simulink model "assignment_R2018A"  (R2018a)
settings: Solver=VariableStepAuto  StartTime=0.0  StopTime=simulation_time
undefined symbols (not defined in the file or in its folder): a, A_BN_0, A_epsilon, A_i, a_m, C_d, dim, DiscIntNeverNeededParam, gm, gn, gsvi, gvali, hm, hn, hsvi, hvali, I, i, I_inv, k_bdot, k_d, k_p, m_max, max_momentum, max_torque, mu, nadir_vector, OMG, omg, phi_0, psi_0, q_0, q_c, R_e, rho_d, rho_s, sigma_e, theta, theta_0, w_0, w_e
libraries: sharedutil x4, simulink_extras x3, aerolibconvert2 x2, simulink x2, vrlib x1
(part 1 of 2)
settings Model: Creator=fcuzzocrea  LastModifiedBy=fcuzzocrea
settings SolverCC: ShapePreserveControl=EnableAll
settings OptimizationCC: DefaultParameterBehavior=Inlined  UseDivisionForNetSlopeComputation=on  UseFloatMulNetSlope=on  InlineInvariantSignals=on  PassReuseOutputArgsAs=Individual arguments  ZeroExternalMemoryAtStartup=off  ZeroInternalMemoryAtStartup=off  NoFixptDivByZeroProtection=on  EfficientFloat2IntCast=on  LifeSpan=1  OptimizeBlockOrder=speed  DifferentSizesBufferReuse=on
settings DebuggingCC: ParameterTunabilityLossMsg=error
settings HardwareCC: ProdBitPerInt=16  ProdBitPerPointer=16  ProdBitPerSizeT=16  ProdBitPerPtrDiffT=16  ProdLargestAtomicFloat=None  ProdWordSize=16  ProdLongLongMode=on  ProdHWDeviceType=STMicroelectronics->ST10/Super10  TargetBitPerLong=64  TargetBitPerPointer=64  TargetBitPerSizeT=64  TargetBitPerPtrDiffT=64  TargetLongLongMode=on  TargetIntDivRoundTo=Zero  TargetEndianess=LittleEndian  TargetWordSize=64  TargetHWDeviceType=MATLAB Host  ProdEqTarget=off
settings SFSimCC: MATLABDynamicMemAlloc=off
settings RTWCC: SystemTargetFile=ert.tlc  TemplateMakefile=ert_default_tmf  GenerateReport=on  RTWUseLocalCustomCode=on  IncludeHyperlinkInReport=on  LaunchReport=on  GenerateTraceInfo=on  GenerateTraceReport=on  GenerateTraceReportSl=on  GenerateTraceReportSf=on  GenerateTraceReportEml=on  GenerateCodeMetricsReport=on
settings CodeAppCC: ForceParamTrailComments=on  IgnoreCustomStorageClasses=off  MaxIdLength=128  OperatorAnnotations=on  SimulinkDataObjDesc=on  SFDataObjDesc=on  CustomSymbolStrGlobalVar=rt$N$M  CustomSymbolStrType=$N$M  CustomSymbolStrFcn=$N$M$F  CustomSymbolStrMacro=$N$M  InsertBlockDesc=on
settings ERTTargetCC: GenerateSampleERTMain=on  IncludeMdlTerminateFcn=off  CombineSignalStateStructs=on  SupportComplex=off  SupportContinuousTime=on  SupportNonInlinedSFcns=on  InlinedParameterPlacement=NonHierarchical  ERTCustomFileTemplate=example_file_process.tlc  ERTFilePackagingFormat=CompactWithDataFile

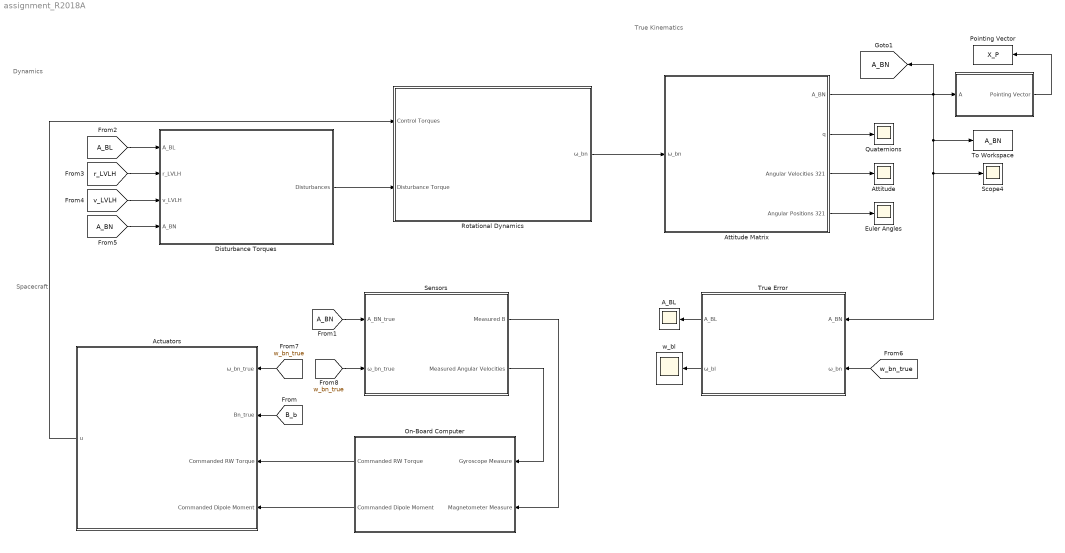
== system assignment_R2018A ==
  note: True Kinematics
  note: Dynamics
  note: Spacecraft
  " " : Subsystem
  " Sensors" : Subsystem
  A_BL : Scope
  Actuators : Subsystem
  Attitude : Scope
  Attitude Matrix : Subsystem
  Disturbance Torques : Subsystem
  Euler Angles : Scope
  On-Board Computer : Subsystem
  Pointing Vector : ToWorkspace  VariableName=X_P  SampleTime=-1
  Quaternions : Scope
  "Rotational Dynamics " : Subsystem
  Scope4 : Scope
  To Workspace : ToWorkspace  VariableName=A_BN  SampleTime=-1
  True Error : Subsystem
  w_bl : Scope
  tag scope: A_BN=global
  wires:
  [r_LVLH] -> Disturbance Torques/2(r_LVLH)
  " "/1("Pointing Vector ") -> Pointing Vector/1
  Attitude Matrix/4(Angular Positions 321) -> Euler Angles/1
  Attitude Matrix/2(q) -> Quaternions/1
  Attitude Matrix/1(A_BN) -> " "/1(A), To Workspace/1, Scope4/1, True Error/1(A_BN), [A_BN]
  [A_BL] -> Disturbance Torques/1(A_BL)
  Attitude Matrix/3(Angular Velocities 321) -> Attitude/1
  [A_BN] -> Disturbance Torques/4(A_BN)
  Disturbance Torques/1(Disturbances) -> "Rotational Dynamics "/2("Disturbance Torque ")
  [v_LVLH] -> Disturbance Torques/3(v_LVLH)
  " Sensors"/2(Measured Angular Velocities) -> On-Board Computer/1(Gyroscope Measure)
  " Sensors"/1(Measured B) -> On-Board Computer/2(Magnetometer Measure)
  True Error/1(A_BL) -> A_BL/1
  On-Board Computer/1(Commanded RW Torque) -> Actuators/3(Commanded RW Torque)
  On-Board Computer/2(Commanded Dipole Moment) -> Actuators/4(Commanded Dipole Moment)
  [B_b] -> Actuators/2(Bn_true)
  "Rotational Dynamics "/1(ω_bn) -> Attitude Matrix/1(ω_bn)
  [A_BN] -> " Sensors"/1(A_BN_true)
  [w_bn_true] -> True Error/2(ω_bn)
  [w_bn_true] -> Actuators/1(ω_bn_true)
  [w_bn_true] -> " Sensors"/2(ω_bn_true)
  Actuators/1(u) -> "Rotational Dynamics "/1(Control Torques)
  True Error/2(ω_bl) -> w_bl/1

== system assignment_R2018A/  ==
  A : Inport
  Constant3 : Constant  Value=[1; 0; 0]  VectorParams1D=off
  Math Function : Math  Operator=transpose  SaturateOnIntegerOverflow=on
  Product1 : Product  Multiplication=Matrix(*)
  "Pointing Vector " : Outport
  wires:
  Constant3/1 -> Product1/2
  Math Function/1 -> Product1/1
  A/1 -> Math Function/1
  Product1/1 -> "Pointing Vector "/1

== system assignment_R2018A/ Sensors ==
  A_BN_true : Inport
  ω_bn_true : Inport  Port=2
  Gyroscope : Subsystem
  Magnetometer : Subsystem
  Zero-Order Hold : ZeroOrderHold  SampleTime=-1
  Zero-Order Hold1 : ZeroOrderHold  SampleTime=-1
  Measured B : Outport
  Measured Angular Velocities : Outport  Port=2
  wires:
  A_BN_true/1 -> Magnetometer/1(A_BN)
  ω_bn_true/1 -> Gyroscope/1(ω_bn)
  Gyroscope/1(Angular Velocities) -> Zero-Order Hold/1
  Magnetometer/1(Magnetic Field) -> Zero-Order Hold1/1
  Zero-Order Hold/1 -> Measured Angular Velocities/1
  Zero-Order Hold1/1 -> Measured B/1

== system assignment_R2018A/Actuators ==
  ω_bn_true : Inport
  Bn_true : Inport  Port=2
  Commanded RW Torque : Inport  Port=3
  Commanded Dipole Moment : Inport  Port=4
  Magnetic Torquers : Subsystem
  Reaction Wheels : Subsystem
  Sum : Sum  Inputs=|++
  To Workspace1 : ToWorkspace  VariableName=control_torque  SampleTime=-1
  u : Outport
  wires:
  Reaction Wheels/1(Control Torque) -> Sum/1
  ω_bn_true/1 -> Reaction Wheels/1(w_bn)
  Commanded RW Torque/1 -> Reaction Wheels/2(Commanded Torque)
  Magnetic Torquers/1(Control Torque) -> Sum/2
  Commanded Dipole Moment/1 -> Magnetic Torquers/2(Commanded Dipole Moment)
  Bn_true/1 -> Magnetic Torquers/1(B)
  Sum/1 -> To Workspace1/1, u/1

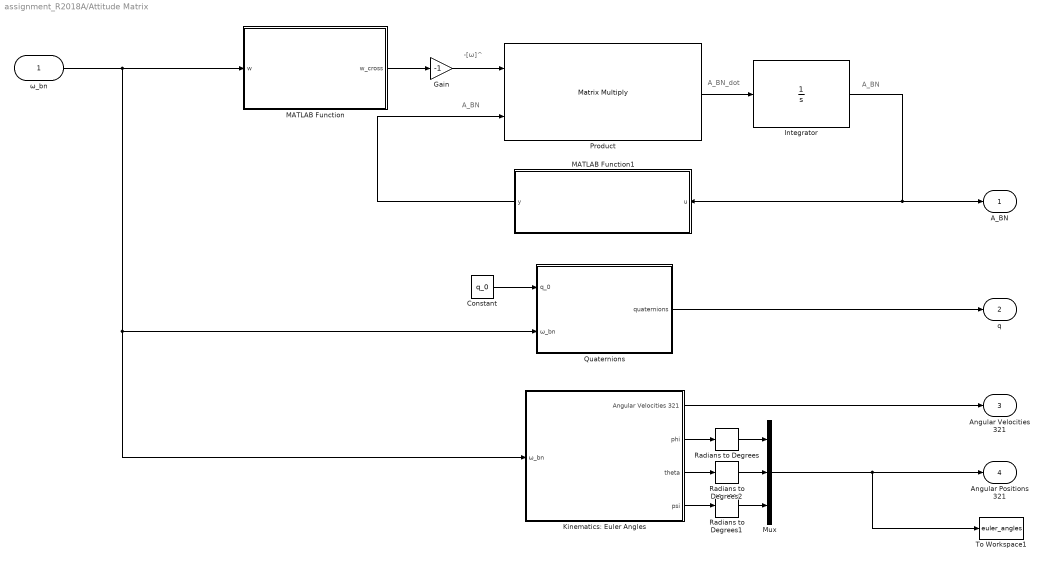
== system assignment_R2018A/Attitude Matrix ==
  note: -[ω]^
  note: A_BN_dot
  note: A_BN
  note: A_BN
  ω_bn : Inport  Unit=rad/s  PortDimensions=3
  Constant : Constant  Value=q_0
  Gain : Gain  Gain=-1
  Integrator : Integrator  InitialCondition=A_BN_0
  Kinematics: Euler Angles : Subsystem
  MATLAB Function : MATLAB Function  TreatAsAtomicUnit=on
  MATLAB Function1 : MATLAB Function  TreatAsAtomicUnit=on
  Mux : Mux  Inputs=3
  Product : Product  Multiplication=Matrix(*)
  Quaternions : Subsystem
  Radians to Degrees : simulink_extras/Transformations/Radians to Degrees
  Radians to Degrees1 : simulink_extras/Transformations/Radians to Degrees
  Radians to Degrees2 : simulink_extras/Transformations/Radians to Degrees
  To Workspace1 : ToWorkspace  VariableName=euler_angles  SampleTime=-1
  A_BN : Outport
  q : Outport  Port=2
  Angular Velocities 321 : Outport  Port=3
  Angular Positions 321 : Outport  Port=4
  wires:
  Product/1 -> Integrator/1
  MATLAB Function/1(w_cross) -> Gain/1
  Integrator/1 -> MATLAB Function1/1(u), A_BN/1
  ω_bn/1 -> MATLAB Function/1(w), Quaternions/2(ω_bn), Kinematics: Euler Angles/1(ω_bn)
  Kinematics: Euler Angles/1(Angular Velocities 321) -> Angular Velocities 321/1
  Kinematics: Euler Angles/3(theta) -> Radians to Degrees2/1
  Kinematics: Euler Angles/4(psi) -> Radians to Degrees1/1
  Kinematics: Euler Angles/2(phi) -> Radians to Degrees/1
  Gain/1 -> Product/1
  Quaternions/1(quaternions) -> q/1
  MATLAB Function1/1(y) -> Product/2
  Constant/1 -> Quaternions/1("q_0 ")
  Radians to Degrees/1 -> Mux/1
  Radians to Degrees2/1 -> Mux/2
  Radians to Degrees1/1 -> Mux/3
  Mux/1 -> To Workspace1/1, Angular Positions 321/1

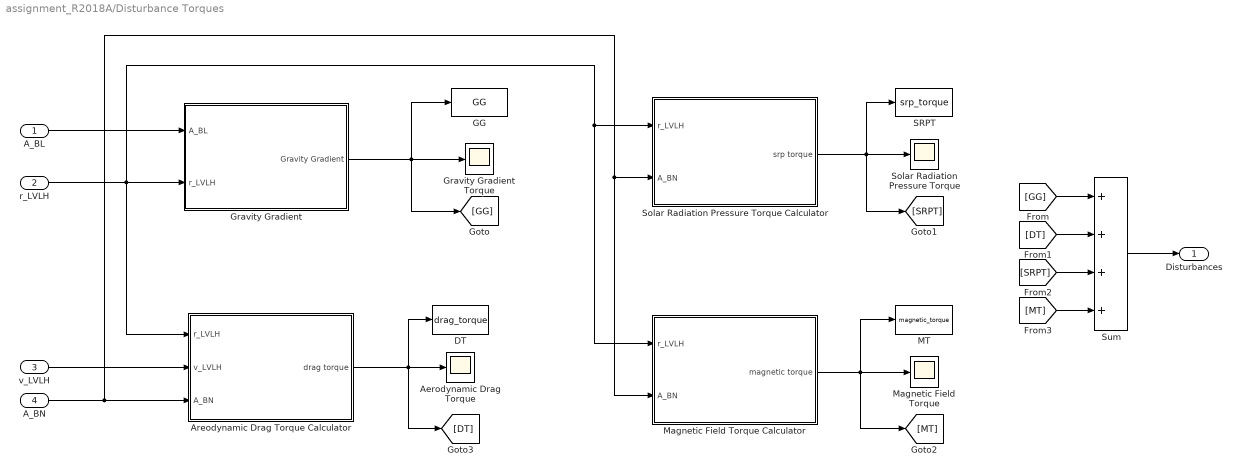
== system assignment_R2018A/Disturbance Torques ==
  A_BL : Inport
  r_LVLH : Inport  Port=2
  v_LVLH : Inport  Port=3
  A_BN : Inport  Port=4
  Aerodynamic Drag Torque : Scope
  "Areodynamic Drag Torque Calculator " : Subsystem
  DT : ToWorkspace  VariableName=drag_torque  SampleTime=-1
  GG : ToWorkspace  VariableName=GG  SampleTime=-1
  Gravity Gradient : Subsystem
  "Gravity Gradient Torque " : Scope
  MT : ToWorkspace  VariableName=magnetic_torque  SampleTime=-1
  Magnetic Field Torque : Scope
  Magnetic Field Torque Calculator : Subsystem
  SRPT : ToWorkspace  VariableName=srp_torque  SampleTime=-1
  Solar Radiation Pressure Torque : Scope
  Solar Radiation Pressure Torque Calculator : Subsystem
  Sum : Sum  Inputs=++++
  Disturbances : Outport
  wires:
  A_BL/1 -> Gravity Gradient/1(A_BL)
  Gravity Gradient/1(Gravity Gradient) -> GG/1, "Gravity Gradient Torque "/1, [GG]
  v_LVLH/1 -> "Areodynamic Drag Torque Calculator "/2(v_LVLH)
  A_BN/1 -> Magnetic Field Torque Calculator/2(A_BN), Solar Radiation Pressure Torque Calculator/2(A_BN), "Areodynamic Drag Torque Calculator "/3(A_BN)
  "Areodynamic Drag Torque Calculator "/1("drag torque ") -> [DT], DT/1, Aerodynamic Drag Torque/1
  Solar Radiation Pressure Torque Calculator/1("srp torque ") -> [SRPT], SRPT/1, Solar Radiation Pressure Torque/1
  Magnetic Field Torque Calculator/1("magnetic torque ") -> MT/1, [MT], Magnetic Field Torque/1
  r_LVLH/1 -> Magnetic Field Torque Calculator/1(r_LVLH), Solar Radiation Pressure Torque Calculator/1(r_LVLH), Gravity Gradient/2(r_LVLH), "Areodynamic Drag Torque Calculator "/1(r_LVLH)
  Sum/1 -> Disturbances/1
  [GG] -> Sum/1
  [DT] -> Sum/2
  [SRPT] -> Sum/3
  [MT] -> Sum/4

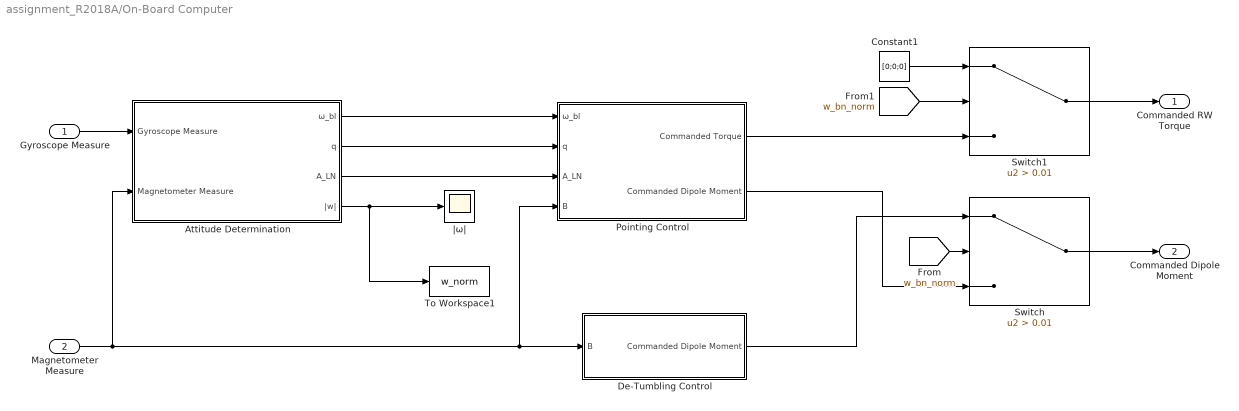
== system assignment_R2018A/On-Board Computer ==
  Gyroscope Measure : Inport
  Magnetometer Measure : Inport  Port=2
  Attitude Determination : Subsystem
  Constant1 : Constant  Value=[0;0;0]
  De-Tumbling Control : Subsystem
  Pointing Control : Subsystem
  Switch : Switch  Criteria=u2 > Threshold  Threshold=0.01
  Switch1 : Switch  Criteria=u2 > Threshold  Threshold=0.01
  To Workspace1 : ToWorkspace  VariableName=w_norm  SampleTime=-1
  |ω| : Scope
  Commanded RW Torque : Outport
  Commanded Dipole Moment : Outport  Port=2
  wires:
  Pointing Control/1(Commanded Torque) -> Switch1/3
  Pointing Control/2(Commanded Dipole Moment) -> Switch/3
  De-Tumbling Control/1(Commanded Dipole Moment) -> Switch/1
  [w_bn_norm] -> Switch/2
  [w_bn_norm] -> Switch1/2
  Switch/1 -> Commanded Dipole Moment/1
  Switch1/1 -> Commanded RW Torque/1
  Constant1/1 -> Switch1/1
  Gyroscope Measure/1 -> Attitude Determination/1(Gyroscope Measure)
  Attitude Determination/2(q) -> Pointing Control/2(q)
  Attitude Determination/3(A_LN) -> Pointing Control/3(A_LN)
  Magnetometer Measure/1 -> Attitude Determination/2(Magnetometer Measure), Pointing Control/4(B), De-Tumbling Control/1(B)
  Attitude Determination/4(|w|) -> To Workspace1/1, |ω|/1
  Attitude Determination/1(ω_bl) -> Pointing Control/1(ω_bl)

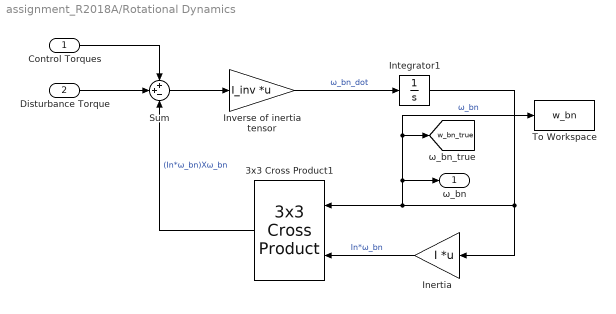
== system assignment_R2018A/Rotational Dynamics  ==
  Control Torques : Inport
  "Disturbance Torque " : Inport  Port=2
  3x3 Cross Product1 : sharedutil/3x3 Cross Product  aMode=aMode
      settings: SourceProductBaseCode=AE
  Inertia : Gain  Gain=I  Multiplication=Matrix(K*u)
  Integrator1 : Integrator  InitialCondition=w_0
  Inverse of inertia tensor : Gain  Gain=I_inv  Multiplication=Matrix(K*u)
  Sum : Sum  Inputs=++-
  To Workspace : ToWorkspace  VariableName=w_bn  SampleTime=-1
  ω_bn : Outport
  tag scope: w_bn_true=global
  wires:
  Inertia/1 -> 3x3 Cross Product1/2  "In*ω_bn"
  Inverse of inertia tensor/1 -> Integrator1/1  "ω_bn_dot"
  3x3 Cross Product1/1 -> Sum/3  "(In*ω_bn)Xω_bn"
  Integrator1/1 -> 3x3 Cross Product1/1, To Workspace/1, [w_bn_true], ω_bn/1, Inertia/1  "ω_bn"
  Sum/1 -> Inverse of inertia tensor/1
  Control Torques/1 -> Sum/1
  "Disturbance Torque "/1 -> Sum/2

== system assignment_R2018A/True Error ==
  A_BN : Inport
  ω_bn : Inport  Port=2
  Angular velocity of the orbital pointing frame : Subsystem
  Attitude Error : Subsystem
  Body\LVLH Difference : Subsystem
  To Workspace : ToWorkspace  VariableName=w_bl  SampleTime=-1
  A_BL : Outport
  ω_bl : Outport  Port=2
  tag scope: A_BL=global
  wires:
  ω_bn/1 -> Attitude Error/1(ω_bn)
  A_BN/1 -> Body\LVLH Difference/1("A_BN ")
  Angular velocity of the orbital pointing frame/1(ω_ln) -> Attitude Error/3("ω_ln ")
  Attitude Error/1(ω_bl) -> To Workspace/1, ω_bl/1
  Body\LVLH Difference/1("A_BL ") -> [A_BL], A_BL/1, Attitude Error/2("A_BL ")

== system assignment_R2018A/ Sensors/Gyroscope ==
  ω_bn : Inport
  Gain : Gain  Gain=sigma_e
  Random Number : RandomNumber  SampleTime=1
  Sum : Sum  Inputs=|++
  Angular Velocities : Outport
  wires:
  ω_bn/1 -> Sum/1
  Random Number/1 -> Gain/1
  Sum/1 -> Angular Velocities/1
  Gain/1 -> Sum/2

== system assignment_R2018A/ Sensors/Magnetometer ==
  A_BN : Inport
  Gain : Gain  Gain=A_epsilon  Multiplication=Matrix(K*u)
  Matrix Multiply : Product  Multiplication=Matrix(*)
  Sum : Sum  Inputs=|++
  Uniform Random Number : UniformRandomNumber  Minimum=5*1e-12  Maximum=1.5*1e-8  SampleTime=1
  Magnetic Field : Outport
  wires:
  Matrix Multiply/1 -> Sum/1
  A_BN/1 -> Matrix Multiply/1
  [B_n] -> Gain/1
  Gain/1 -> Matrix Multiply/2
  Uniform Random Number/1 -> Sum/2
  Sum/1 -> Magnetic Field/1

== system assignment_R2018A/Actuators/Magnetic Torquers ==
  note: m
  B : Inport
  Commanded Dipole Moment : Inport  Port=2
  3x3 Cross Product1 : sharedutil/3x3 Cross Product  aMode=aMode
      settings: SourceProductBaseCode=AE
  Saturation : Saturate  UpperLimit=m_max  LowerLimit=-m_max
  Control Torque : Outport
  wires:
  B/1 -> 3x3 Cross Product1/2
  3x3 Cross Product1/1 -> Control Torque/1
  Commanded Dipole Moment/1 -> Saturation/1
  Saturation/1 -> 3x3 Cross Product1/1

== system assignment_R2018A/Actuators/Reaction Wheels ==
  w_bn : Inport
  Commanded Torque : Inport  Port=2
  Integrator : Integrator  InitialCondition=[0,0,0]  UpperSaturationLimit=max_momentum  LowerSaturationLimit=-max_momentum
  "Reaction Wheels Dynamics " : Subsystem
  Saturation : Saturate  UpperLimit=max_torque  LowerLimit=-max_torque
  Saturation1 : Saturate  UpperLimit=max_momentum  LowerLimit=-max_momentum
  Control Torque : Outport
  wires:
  "Reaction Wheels Dynamics "/1(u) -> Control Torque/1
  w_bn/1 -> "Reaction Wheels Dynamics "/1(w_bn)
  Commanded Torque/1 -> Saturation/1
  Integrator/1 -> Saturation1/1
  Saturation/1 -> Integrator/1, "Reaction Wheels Dynamics "/2(h_d_dot)
  Saturation1/1 -> "Reaction Wheels Dynamics "/3(h_d)

== system assignment_R2018A/Attitude Matrix/Kinematics: Euler Angles ==
  ω_bn : Inport
  Integrator : Integrator  InitialCondition=phi_0
  Integrator1 : Integrator  InitialCondition=theta_0
  Integrator2 : Integrator  InitialCondition=psi_0
  MATLAB Function : MATLAB Function  TreatAsAtomicUnit=on
  Mux : Mux  Inputs=3
  Angular Velocities 321 : Outport
  phi : Outport  Port=2
  theta : Outport  Port=3
  psi : Outport  Port=4
  wires:
  Integrator2/1 -> MATLAB Function/3(psi), Mux/3, psi/1
  Mux/1 -> Angular Velocities 321/1
  Integrator1/1 -> MATLAB Function/2(tetha), Mux/2, theta/1
  Integrator/1 -> Mux/1, phi/1
  MATLAB Function/3(psi_dot) -> Integrator2/1
  MATLAB Function/2(tetha_dot) -> Integrator1/1
  MATLAB Function/1(phi_dot) -> Integrator/1
  ω_bn/1 -> MATLAB Function/1(w)

== system assignment_R2018A/Attitude Matrix/Quaternions ==
  "q_0 " : Inport
  ω_bn : Inport  Port=2
  Integrator2 : Integrator  InitialConditionSource=external  InitialCondition=q_0
  Quaternion Kinematics : MATLAB Function  TreatAsAtomicUnit=on
  quaternions : Outport
  wires:
  Integrator2/1 -> Quaternion Kinematics/1(q), quaternions/1  "q"
  Quaternion Kinematics/1(q_dot) -> Integrator2/1  "dq"
  ω_bn/1 -> Quaternion Kinematics/2(omega)  "ω_b"
  "q_0 "/1 -> Integrator2/2

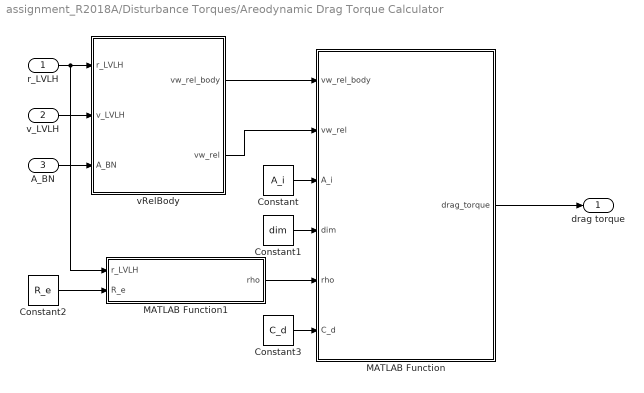
== system assignment_R2018A/Disturbance Torques/Areodynamic Drag Torque Calculator  ==
  r_LVLH : Inport
  v_LVLH : Inport  Port=2
  A_BN : Inport  Port=3
  Constant : Constant  Value=A_i
  Constant1 : Constant  Value=dim
  Constant2 : Constant  Value=R_e
  Constant3 : Constant  Value=C_d
  MATLAB Function : MATLAB Function  TreatAsAtomicUnit=on
  MATLAB Function1 : MATLAB Function  TreatAsAtomicUnit=on
  vRelBody : Subsystem
  "drag torque " : Outport
  wires:
  r_LVLH/1 -> MATLAB Function1/1(r_LVLH), vRelBody/1(r_LVLH)
  v_LVLH/1 -> vRelBody/2(v_LVLH)
  A_BN/1 -> vRelBody/3(A_BN)
  vRelBody/1(vw_rel_body) -> MATLAB Function/1(vw_rel_body)
  Constant/1 -> MATLAB Function/3(A_i)
  Constant1/1 -> MATLAB Function/4(dim)
  Constant3/1 -> MATLAB Function/6(C_d)
  Constant2/1 -> MATLAB Function1/2(R_e)
  MATLAB Function1/1(rho) -> MATLAB Function/5(rho)
  MATLAB Function/1(drag_torque) -> "drag torque "/1
  vRelBody/2(vw_rel) -> MATLAB Function/2(vw_rel)

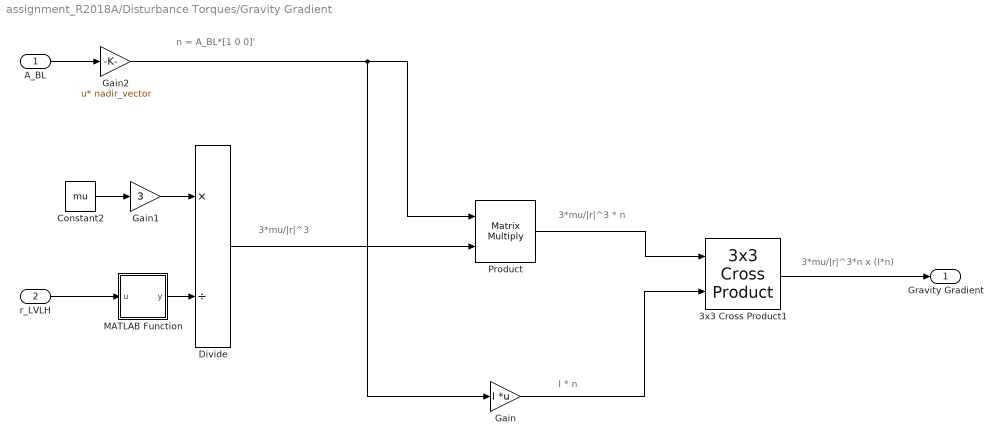
== system assignment_R2018A/Disturbance Torques/Gravity Gradient ==
  note: 3*mu/|r|^3*n x (I*n)
  note: I * n
  note: 3*mu/|r|^3 * n
  note: n = A_BL*[1 0 0]'
  note: 3*mu/|r|^3
  A_BL : Inport
  r_LVLH : Inport  Port=2
  3x3 Cross Product1 : sharedutil/3x3 Cross Product  aMode=aMode
      settings: SourceProductBaseCode=AE
  Constant2 : Constant  Value=mu
  Divide : Product  Inputs=*/
  Gain : Gain  Gain=I  Multiplication=Matrix(K*u)
  Gain1 : Gain  Gain=3
  Gain2 : Gain  Gain=nadir_vector  Multiplication=Matrix(u*K)
  MATLAB Function : MATLAB Function  TreatAsAtomicUnit=on
  Product : Product  Multiplication=Matrix(*)
  Gravity Gradient : Outport
  wires:
  A_BL/1 -> Gain2/1
  r_LVLH/1 -> MATLAB Function/1(u)
  Constant2/1 -> Gain1/1
  Divide/1 -> Product/2
  Product/1 -> 3x3 Cross Product1/1
  Gain/1 -> 3x3 Cross Product1/2
  Gain2/1 -> Gain/1, Product/1
  3x3 Cross Product1/1 -> Gravity Gradient/1
  Gain1/1 -> Divide/1
  MATLAB Function/1(y) -> Divide/2

== system assignment_R2018A/Disturbance Torques/Magnetic Field Torque Calculator ==
  r_LVLH : Inport
  A_BN : Inport  Port=2
  3x3 Cross Product : sharedutil/3x3 Cross Product  aMode=aMode
      settings: SourceProductBaseCode=AE
  Complete Model : Subsystem
  "Spacecraft " : Subsystem
  "magnetic torque " : Outport
  wires:
  r_LVLH/1 -> Complete Model/2(r_LVLH)
  A_BN/1 -> Complete Model/1(A_BN)
  3x3 Cross Product/1 -> "magnetic torque "/1
  Complete Model/1(B) -> 3x3 Cross Product/2
  "Spacecraft "/1(m) -> 3x3 Cross Product/1

== system assignment_R2018A/Disturbance Torques/Solar Radiation Pressure Torque Calculator ==
  r_LVLH : Inport
  A_BN : Inport  Port=2
  Constant : Constant  Value=A_i
  Constant1 : Constant  Value=dim
  Constant2 : Constant  Value=rho_s
  Constant3 : Constant  Value=rho_d
  Constant7 : Constant  Value=R_e
  MATLAB Function : MATLAB Function  TreatAsAtomicUnit=on
  Subsystem : Subsystem
  "srp torque " : Outport
  wires:
  A_BN/1 -> Subsystem/1(A_BN)
  Constant/1 -> MATLAB Function/5(A_i)
  Constant1/1 -> MATLAB Function/6(dim)
  Constant3/1 -> MATLAB Function/7(rho_d)
  Constant2/1 -> MATLAB Function/8(rho_s)
  r_LVLH/1 -> Subsystem/2(r_LVLH), MATLAB Function/1(r)
  Constant7/1 -> MATLAB Function/2(R_e)
  MATLAB Function/1(srp_torque) -> "srp torque "/1
  Subsystem/1("S_b ") -> MATLAB Function/3(S_b)
  Subsystem/2(S_eartSun) -> MATLAB Function/4(S_earthSun)

== system assignment_R2018A/On-Board Computer/Attitude Determination ==
  Gyroscope Measure : Inport
  Magnetometer Measure : Inport  Port=2
  Kinematics : Subsystem
  ω norm : Subsystem
  ω_bl : Outport
  q : Outport  Port=2
  A_LN : Outport  Port=3
  |w| : Outport  Port=4
  wires:
  ω norm/1(|ω_bn|) -> |w|/1
  Kinematics/1(ω_bl) -> ω_bl/1
  Gyroscope Measure/1 -> Kinematics/1(Gyroscope Measure), ω norm/1(ω_bn)
  Kinematics/2(q) -> q/1
  Kinematics/3(A_LN) -> A_LN/1
  Magnetometer Measure/1 -> Kinematics/2(Magnetometer Measure)

== system assignment_R2018A/On-Board Computer/De-Tumbling Control ==
  note: m
  B : Inport
  Discrete Derivative1 : simulink/Discrete/Discrete Derivative  gainval=1  ICPrevScaledInput=0.0  OutMin=[]  OutMax=[]  OutDataType=fixdt(1, 16)  OutScaling=2^-10  DoSatur=off
  Divide : Product  Inputs=*/
  Gain1 : Gain  Gain=k_bdot
  MATLAB Function1 : MATLAB Function  TreatAsAtomicUnit=on
  Commanded Dipole Moment : Outport
  wires:
  B/1 -> MATLAB Function1/1(u), Discrete Derivative1/1
  MATLAB Function1/1(y) -> Divide/2
  Gain1/1 -> Divide/1
  Discrete Derivative1/1 -> Gain1/1
  Divide/1 -> Commanded Dipole Moment/1

== system assignment_R2018A/On-Board Computer/Pointing Control ==
  ω_bl : Inport
  q : Inport  Port=2
  A_LN : Inport  Port=3
  B : Inport  Port=4
  Mixer : Subsystem
  Quaternion Feedback Control : Subsystem
  Commanded Torque : Outport
  Commanded Dipole Moment : Outport  Port=2
  wires:
  ω_bl/1 -> Quaternion Feedback Control/1(ω_bl)
  q/1 -> Quaternion Feedback Control/2(q)
  Quaternion Feedback Control/1(u_id) -> Mixer/1(u_id)
  Mixer/1(Commanded Torque) -> Commanded Torque/1
  Mixer/2("Commanded Dipole Moment ") -> Commanded Dipole Moment/1
  B/1 -> Mixer/2(B)
  A_LN/1 -> Quaternion Feedback Control/3(A_LN)

== system assignment_R2018A/True Error/Angular velocity of the orbital pointing frame ==
  Derivative : Derivative
  Gain : Gain  Gain=-1
  MATLAB Function : MATLAB Function  TreatAsAtomicUnit=on
  Math Function : Math  Operator=transpose  SaturateOnIntegerOverflow=on
  Product : Product  Multiplication=Matrix(*)
  To Workspace : ToWorkspace  VariableName=w_ln  SampleTime=-1
  ω_ln : Outport
  wires:
  Math Function/1 -> Product/2
  Product/1 -> MATLAB Function/1(w_ln_cross)
  [A_LN] -> Math Function/1, Gain/1
  Gain/1 -> Derivative/1
  MATLAB Function/1(w_ln) -> To Workspace/1, ω_ln/1
  Derivative/1 -> Product/1

== system assignment_R2018A/True Error/Attitude Error ==
  ω_bn : Inport
  "A_BL " : Inport  Port=2
  "ω_ln " : Inport  Port=3
  Product : Product  Multiplication=Matrix(*)
  Subtract : Sum  Inputs=+-
  ω_bl : Outport
  wires:
  Product/1 -> Subtract/2
  Subtract/1 -> ω_bl/1
  ω_bn/1 -> Subtract/1
  "A_BL "/1 -> Product/1
  "ω_ln "/1 -> Product/2

== system assignment_R2018A/True Error/Body\LVLH Difference ==
  "A_BN " : Inport
  LVLH : Subsystem
  Math Function1 : Math  Operator=transpose  SaturateOnIntegerOverflow=on
  Product : Product  Multiplication=Matrix(*)
  Scope : Scope
  Scope1 : Scope
  "A_BL " : Outport
  wires:
  "A_BN "/1 -> Scope/1, Product/1
  Product/1 -> "A_BL "/1
  Math Function1/1 -> Product/2
  LVLH/1("A_LN ") -> Scope1/1, Math Function1/1

== system assignment_R2018A/Actuators/Reaction Wheels/Reaction Wheels Dynamics  ==
  w_bn : Inport
  h_d_dot : Inport  Port=2
  h_d : Inport  Port=3
  Gain : Gain  Gain=-1
  MATLAB Function : MATLAB Function  TreatAsAtomicUnit=on
  u : Outport
  wires:
  MATLAB Function/1(u) -> Gain/1
  w_bn/1 -> MATLAB Function/3(w_bn)
  h_d_dot/1 -> MATLAB Function/1(h_d_dot)
  h_d/1 -> MATLAB Function/2(h_d)
  Gain/1 -> u/1

== system assignment_R2018A/Disturbance Torques/Areodynamic Drag Torque Calculator /vRelBody ==
  r_LVLH : Inport
  v_LVLH : Inport  Port=2
  A_BN : Inport  Port=3
  Add : Sum
  Constant : Constant  Value=w_e
  Cross Product : vrlib/Utilities/Cross Product
      settings: SourceProductBaseCode=VR
  Product : Product  Multiplication=Matrix(*)
  vw_rel_body : Outport
  vw_rel : Outport  Port=2
  wires:
  Add/1 -> vw_rel/1, Product/2
  Constant/1 -> Cross Product/1
  r_LVLH/1 -> Cross Product/2
  Product/1 -> vw_rel_body/1
  v_LVLH/1 -> Add/1
  A_BN/1 -> Product/1
  Cross Product/1 -> Add/2

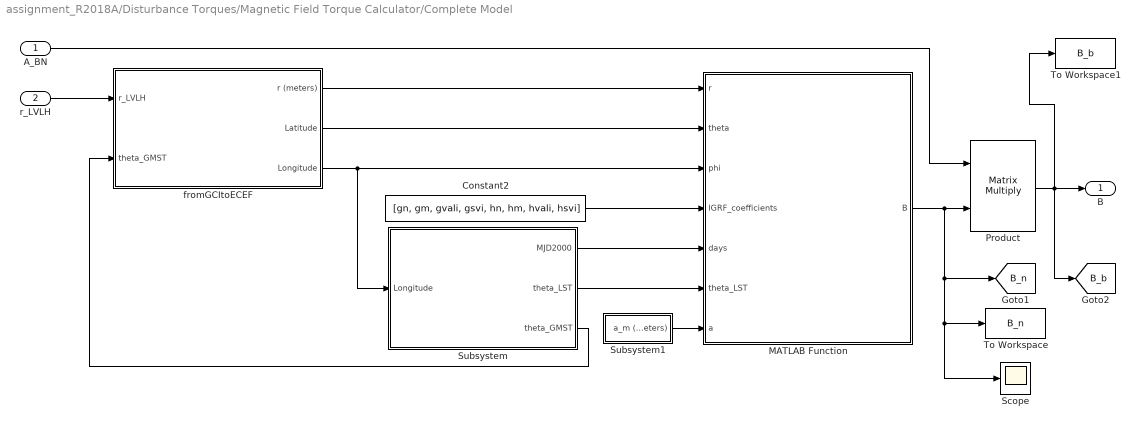
== system assignment_R2018A/Disturbance Torques/Magnetic Field Torque Calculator/Complete Model ==
  A_BN : Inport
  r_LVLH : Inport  Port=2
  Constant2 : Constant  Value="[gn, gm, gvali,  gsvi, hn,  hm,  hvali,  hsvi]"
  MATLAB Function : MATLAB Function  TreatAsAtomicUnit=on
  Product : Product  Multiplication=Matrix(*)
  Scope : Scope
  Subsystem : Subsystem
  Subsystem1 : Subsystem
  To Workspace : ToWorkspace  VariableName=B_n  SampleTime=-1
  To Workspace1 : ToWorkspace  VariableName=B_b  SampleTime=-1
  fromGCItoECEF : Subsystem
  B : Outport
  tag scope: B_b=global, B_n=global
  wires:
  Subsystem/3(theta_GMST) -> fromGCItoECEF/2(theta_GMST)
  fromGCItoECEF/3(Longitude) -> MATLAB Function/3(phi), Subsystem/1(Longitude)
  Subsystem/1(MJD2000) -> MATLAB Function/5(days)
  r_LVLH/1 -> fromGCItoECEF/1(r_LVLH)
  fromGCItoECEF/2(Latitude) -> MATLAB Function/2(theta)
  Subsystem/2(theta_LST) -> MATLAB Function/6(theta_LST)
  fromGCItoECEF/1(r (meters)) -> MATLAB Function/1(r)
  A_BN/1 -> Product/1
  Product/1 -> [B_b], To Workspace1/1, B/1
  Constant2/1 -> MATLAB Function/4(IGRF_coefficients)
  Subsystem1/1(a_m (meters)) -> MATLAB Function/7(a)
  MATLAB Function/1(B) -> Product/2, To Workspace/1, Scope/1, [B_n]

== system assignment_R2018A/Disturbance Torques/Magnetic Field Torque Calculator/Spacecraft  ==
  Constant2 : Constant  Value=0.1
  Vector Concatenate : Concatenate  NumInputs=3
  m : Outport
  wires:
  Vector Concatenate/1 -> m/1
  Constant2/1 -> Vector Concatenate/1, Vector Concatenate/3, Vector Concatenate/2

== system assignment_R2018A/Disturbance Torques/Solar Radiation Pressure Torque Calculator/Subsystem ==
  A_BN : Inport
  r_LVLH : Inport  Port=2
  Clock : Clock
  Julian Date Conversion : aerolibconvert2/Julian Date Conversion  year=2019  month=January  day=1  hour=12  min=0  sec=0  modflag=off  deltaT=Sec  errorflag=Error
      settings: SourceProductName=Aerospace Blockset  SourceProductBaseCode=AE
  Product2 : Product  Multiplication=Matrix(*)
  sunPosition : MATLAB Function  TreatAsAtomicUnit=on
  "S_b " : Outport
  S_eartSun : Outport  Port=2
  wires:
  Clock/1 -> Julian Date Conversion/1
  Julian Date Conversion/1 -> sunPosition/1(JD)
  Product2/1 -> "S_b "/1
  sunPosition/1(S_i) -> Product2/2
  A_BN/1 -> Product2/1
  r_LVLH/1 -> sunPosition/2(r_LVLH)
  sunPosition/2(S_eartSun) -> S_eartSun/1

== system assignment_R2018A/On-Board Computer/Attitude Determination/Kinematics ==
  Gyroscope Measure : Inport
  Magnetometer Measure : Inport  Port=2
  " " : Subsystem
  "Error on ω " : Subsystem
  LVLH : Subsystem
  Quaternions : Subsystem
  ω_bl : Outport
  q : Outport  Port=2
  A_LN : Outport  Port=3
  wires:
  Quaternions/2(q) -> q/1
  " "/1(ω_ln) -> "Error on ω "/2("ω_ln ")
  "Error on ω "/1(ω_bl) -> ω_bl/1
  Gyroscope Measure/1 -> Quaternions/1(Angular Velocities), "Error on ω "/1(ω_bn)
  Quaternions/1(A_BN) -> "Error on ω "/4("A_BN ")
  LVLH/1("A_LN ") -> " "/1(A_LN), "Error on ω "/3(A_LN), A_LN/1
  Magnetometer Measure/1 -> Quaternions/2(Magnetometer Measure)

== system assignment_R2018A/On-Board Computer/Attitude Determination/ω norm ==
  ω_bn : Inport
  MATLAB Function1 : MATLAB Function  TreatAsAtomicUnit=on
  |ω_bn| : Outport
  tag scope: w_bn_norm=global
  wires:
  MATLAB Function1/1(y) -> [w_bn_norm], |ω_bn|/1
  ω_bn/1 -> MATLAB Function1/1(u)

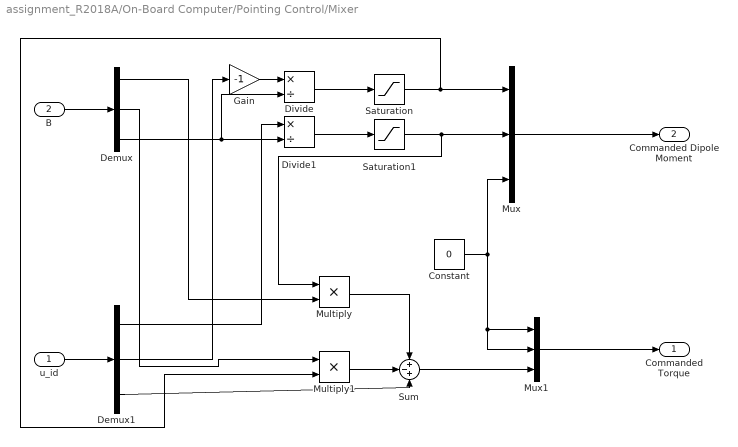
== system assignment_R2018A/On-Board Computer/Pointing Control/Mixer ==
  u_id : Inport
  B : Inport  Port=2
  Constant : Constant  Value=0
  Demux : Demux  Outputs=3
  Demux1 : Demux  Outputs=3
  Divide : Product  Inputs=*/
  Divide1 : Product  Inputs=*/
  Gain : Gain  Gain=-1
  Multiply : Product
  Multiply1 : Product
  Mux : Mux  Inputs=3
  Mux1 : Mux  Inputs=3
  Saturation : Saturate  UpperLimit=m_max  LowerLimit=-m_max
  Saturation1 : Saturate  UpperLimit=m_max  LowerLimit=-m_max
  Sum : Sum  Inputs=+-+
  Commanded Torque : Outport
  "Commanded Dipole Moment " : Outport  Port=2
  wires:
  u_id/1 -> Demux1/1
  Demux1/2 -> Gain/1
  Gain/1 -> Divide/1
  Demux1/1 -> Divide1/1
  Multiply/1 -> Sum/1
  Demux1/3 -> Sum/3
  Multiply1/1 -> Sum/2
  Demux/1 -> Multiply/2
  Demux/2 -> Multiply1/1
  Sum/1 -> Mux1/3
  Mux/1 -> "Commanded Dipole Moment "/1
  Mux1/1 -> Commanded Torque/1
  B/1 -> Demux/1
  Divide/1 -> Saturation/1
  Divide1/1 -> Saturation1/1
  Constant/1 -> Mux1/2, Mux1/1, Mux/3
  Saturation/1 -> Multiply1/2, Mux/1
  Saturation1/1 -> Multiply/1, Mux/2
  Demux/3 -> Divide1/2, Divide/2

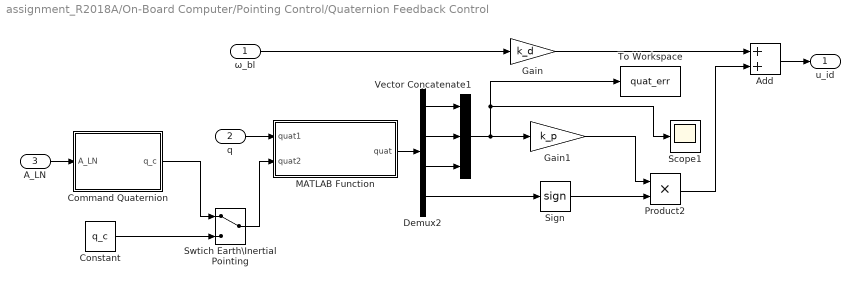
== system assignment_R2018A/On-Board Computer/Pointing Control/Quaternion Feedback Control ==
  ω_bl : Inport
  q : Inport  Port=2
  A_LN : Inport  Port=3
  Add : Sum
  Command Quaternion : Subsystem
  Constant : Constant  Value=q_c
  Demux2 : Demux
  Gain : Gain  Gain=k_d
  Gain1 : Gain  Gain=k_p
  MATLAB Function : MATLAB Function  TreatAsAtomicUnit=on
  Product2 : Product
  Scope1 : Scope
  Sign : Signum
  "Swtich Earth\\Inertial Pointing " : ManualSwitch
  To Workspace : ToWorkspace  VariableName=quat_err  SampleTime=-1
  Vector Concatenate1 : Concatenate  NumInputs=3
  u_id : Outport
  wires:
  Demux2/3 -> Vector Concatenate1/3
  Add/1 -> u_id/1
  ω_bl/1 -> Gain/1
  Demux2/2 -> Vector Concatenate1/2
  Gain/1 -> Add/1
  Demux2/1 -> Vector Concatenate1/1
  Vector Concatenate1/1 -> To Workspace/1, Scope1/1, Gain1/1
  q/1 -> MATLAB Function/1(quat1)
  Gain1/1 -> Product2/1
  Demux2/4 -> Sign/1
  Sign/1 -> Product2/2
  MATLAB Function/1(quat) -> Demux2/1
  A_LN/1 -> Command Quaternion/1(A_LN)
  Command Quaternion/1(q_c) -> "Swtich Earth\\Inertial Pointing "/1
  "Swtich Earth\\Inertial Pointing "/1 -> MATLAB Function/2(quat2)
  Constant/1 -> "Swtich Earth\\Inertial Pointing "/2
  Product2/1 -> Add/2

== system assignment_R2018A/True Error/Body\LVLH Difference/LVLH ==
  Full Orbital Dynamics : Subsystem
  Initial Conditions (KEP) : Constant  Value=[a, e, i, OMG, omg, theta]
  Planetary Constant : Constant  Value=mu
  "A_LN " : Outport
  tag scope: A_LN=global
  wires:
  Planetary Constant/1 -> Full Orbital Dynamics/1(mu)
  Initial Conditions (KEP)/1 -> Full Orbital Dynamics/2(Initial Condition (kep))
  Full Orbital Dynamics/1(A_LN) -> [A_LN], "A_LN "/1

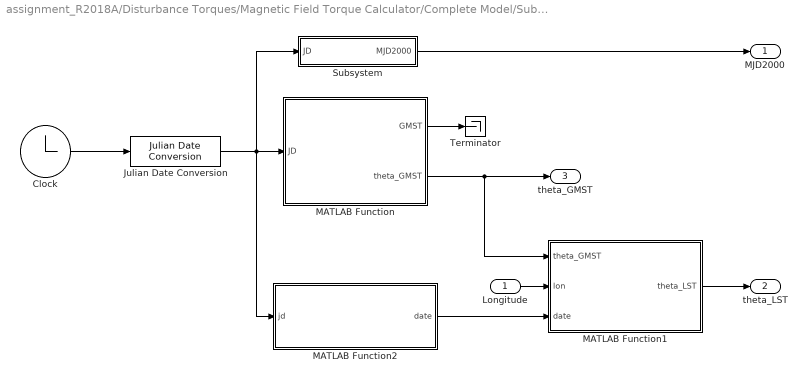
== system assignment_R2018A/Disturbance Torques/Magnetic Field Torque Calculator/Complete Model/Subsystem ==
  Longitude : Inport
  Clock : Clock
  Julian Date Conversion : aerolibconvert2/Julian Date Conversion  year=2019  month=January  day=1  hour=12  min=0  sec=0  modflag=off  deltaT=Sec  errorflag=Error
      settings: SourceProductName=Aerospace Blockset  SourceProductBaseCode=AE
  MATLAB Function : MATLAB Function  TreatAsAtomicUnit=on
  MATLAB Function1 : MATLAB Function  TreatAsAtomicUnit=on
  MATLAB Function2 : MATLAB Function  TreatAsAtomicUnit=on
  Subsystem : Subsystem
  Terminator : Terminator
  MJD2000 : Outport
  theta_LST : Outport  Port=2
  theta_GMST : Outport  Port=3
  wires:
  Clock/1 -> Julian Date Conversion/1
  Julian Date Conversion/1 -> MATLAB Function2/1(jd), Subsystem/1(JD), MATLAB Function/1(JD)
  Subsystem/1(MJD2000) -> MJD2000/1
  MATLAB Function/2(theta_GMST) -> MATLAB Function1/1(theta_GMST), theta_GMST/1
  MATLAB Function/1(GMST) -> Terminator/1
  Longitude/1 -> MATLAB Function1/2(lon)
  MATLAB Function1/1(theta_LST) -> theta_LST/1
  MATLAB Function2/1(date) -> MATLAB Function1/3(date)

== system assignment_R2018A/Disturbance Torques/Magnetic Field Torque Calculator/Complete Model/Subsystem1 ==
  Constant : Constant  Value=a_m
  Product4 : Product
  meters : Constant  Value=1000
  a_m (meters) : Outport
  wires:
  Constant/1 -> Product4/1
  meters/1 -> Product4/2
  Product4/1 -> a_m (meters)/1

== system assignment_R2018A/Disturbance Torques/Magnetic Field Torque Calculator/Complete Model/fromGCItoECEF ==
  r_LVLH : Inport
  theta_GMST : Inport  Port=2
  MATLAB Function1 : MATLAB Function  TreatAsAtomicUnit=on
  Product4 : Product
  meters : Constant  Value=1000
  r (meters) : Outport
  Latitude : Outport  Port=2
  Longitude : Outport  Port=3
  wires:
  MATLAB Function1/2(lat) -> Latitude/1
  theta_GMST/1 -> MATLAB Function1/2(theta_GMST)
  MATLAB Function1/1(r) -> Product4/2
  Product4/1 -> r (meters)/1
  MATLAB Function1/3(lon) -> Longitude/1
  r_LVLH/1 -> MATLAB Function1/1(r_LVLH)
  meters/1 -> Product4/1

== system assignment_R2018A/On-Board Computer/Attitude Determination/Kinematics/  ==
  A_LN : Inport
  Discrete Derivative : simulink/Discrete/Discrete Derivative  gainval=1.0  ICPrevScaledInput=0.0  OutMin=[]  OutMax=[]  OutDataType=fixdt(1, 16)  OutScaling=2^-10  DoSatur=off
  Gain : Gain  Gain=-1
  MATLAB Function : MATLAB Function  TreatAsAtomicUnit=on
  Math Function : Math  Operator=transpose  SaturateOnIntegerOverflow=on
  Product : Product  Multiplication=Matrix(*)
  ω_ln : Outport
  wires:
  Math Function/1 -> Product/2
  Product/1 -> MATLAB Function/1(w_ln_cross)
  A_LN/1 -> Math Function/1, Gain/1
  Gain/1 -> Discrete Derivative/1
  MATLAB Function/1(w_ln) -> ω_ln/1
  Discrete Derivative/1 -> Product/1

== system assignment_R2018A/On-Board Computer/Attitude Determination/Kinematics/Error on ω  ==
  note: A_BL
  ω_bn : Inport
  "ω_ln " : Inport  Port=2
  A_LN : Inport  Port=3
  "A_BN " : Inport  Port=4
  A_BL : Scope
  Math Function1 : Math  Operator=transpose  SaturateOnIntegerOverflow=on
  Product : Product  Multiplication=Matrix(*)
  Product1 : Product  Multiplication=Matrix(*)
  Subtract : Sum  Inputs=+-
  ω_bl : Outport
  wires:
  Subtract/1 -> ω_bl/1
  ω_bn/1 -> Subtract/1
  "ω_ln "/1 -> Product/2
  Product/1 -> Subtract/2
  A_LN/1 -> Math Function1/1
  Math Function1/1 -> Product1/2
  "A_BN "/1 -> Product1/1
  Product1/1 -> A_BL/1, Product/1

== system assignment_R2018A/On-Board Computer/Attitude Determination/Kinematics/LVLH ==
  Full Orbital Dynamics : Subsystem
  Initial Conditions (KEP) : Constant  Value=[a, e, i, OMG, omg, theta]
  Planetary Constant : Constant  Value=mu
  "A_LN " : Outport
  wires:
  Planetary Constant/1 -> Full Orbital Dynamics/1(mu)
  Initial Conditions (KEP)/1 -> Full Orbital Dynamics/2(Initial Condition (kep))
  Full Orbital Dynamics/1(A_LN) -> "A_LN "/1

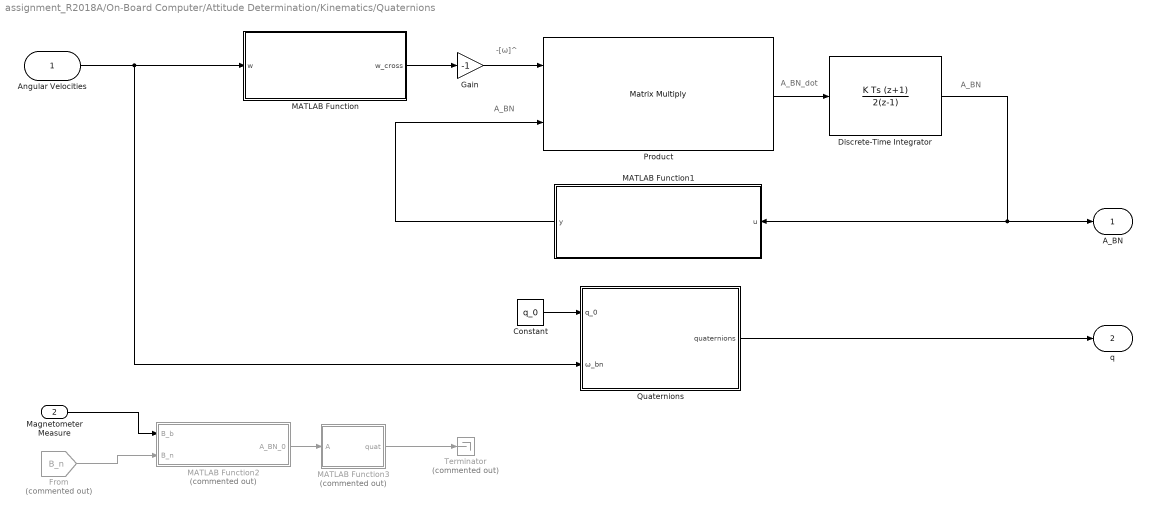
== system assignment_R2018A/On-Board Computer/Attitude Determination/Kinematics/Quaternions ==
  note: A_BN_dot
  note: -[ω]^
  note: A_BN
  note: A_BN
  Angular Velocities : Inport  Unit=rad/s  PortDimensions=3
  Magnetometer Measure : Inport  Port=2
  Constant : Constant  Value=q_0
  Discrete-Time Integrator : DiscreteIntegrator  IntegratorMethod=Integration: Trapezoidal  InitialCondition=A_BN_0  SampleTime=-1  ICPrevOutput=DiscIntNeverNeededParam  ICPrevScaledInput=DiscIntNeverNeededParam
  From : From  Commented=on  GotoTag=B_n  TagVisibility=global
  Gain : Gain  Gain=-1
  MATLAB Function : MATLAB Function  TreatAsAtomicUnit=on
  MATLAB Function1 : MATLAB Function  TreatAsAtomicUnit=on
  MATLAB Function2 : MATLAB Function  Commented=on  TreatAsAtomicUnit=on
  MATLAB Function3 : MATLAB Function  Commented=on  TreatAsAtomicUnit=on
  Product : Product  Multiplication=Matrix(*)
  Quaternions : Subsystem
  Terminator : Terminator  Commented=on
  A_BN : Outport
  q : Outport  Port=2
  wires:
  Product/1 -> Discrete-Time Integrator/1
  MATLAB Function1/1(y) -> Product/2
  Discrete-Time Integrator/1 -> A_BN/1, MATLAB Function1/1(u)
  Angular Velocities/1 -> Quaternions/2(ω_bn), MATLAB Function/1(w)
  MATLAB Function/1(w_cross) -> Gain/1
  Gain/1 -> Product/1
  Quaternions/1(quaternions) -> q/1
  Constant/1 -> Quaternions/1("q_0 ")
  Magnetometer Measure/1 -> MATLAB Function2/1(B_b)
  From/1 -> MATLAB Function2/2(B_n)
  MATLAB Function2/1(A_BN_0) -> MATLAB Function3/1(A)
  MATLAB Function3/1(quat) -> Terminator/1

== system assignment_R2018A/On-Board Computer/Pointing Control/Quaternion Feedback Control/Command Quaternion ==
  A_LN : Inport
  MATLAB Function : MATLAB Function  TreatAsAtomicUnit=on
  MATLAB Function1 : MATLAB Function  TreatAsAtomicUnit=on
  q_c : Outport
  wires:
  MATLAB Function/1(quat) -> MATLAB Function1/1(quat)
  MATLAB Function1/1(qInv) -> q_c/1
  A_LN/1 -> MATLAB Function/1(A)

== system assignment_R2018A/True Error/Body\LVLH Difference/LVLH/Full Orbital Dynamics ==
  mu : Inport
  Initial Condition (kep) : Inport  Port=2
  " " : ToWorkspace  VariableName=r_LVLH  SampleTime=-1
  Compute R and V of reference orbit : Subsystem
  MATLAB Function : MATLAB Function  TreatAsAtomicUnit=on
  To Workspace : ToWorkspace  VariableName=A_LN  SampleTime=-1
  A_LN : Outport
  tag scope: r_LVLH=global, v_LVLH=global
  wires:
  mu/1 -> Compute R and V of reference orbit/1(mu)
  Initial Condition (kep)/1 -> Compute R and V of reference orbit/2(Initial Conditions)
  Compute R and V of reference orbit/1(r) -> [r_LVLH], " "/1, MATLAB Function/1(r)
  MATLAB Function/1(A_LN) -> A_LN/1, To Workspace/1
  Compute R and V of reference orbit/2(r_dot) -> [v_LVLH], MATLAB Function/2(r_dot)

== system assignment_R2018A/Disturbance Torques/Magnetic Field Torque Calculator/Complete Model/Subsystem/Subsystem ==
  JD : Inport
  Constant1 : Constant  Value=2400000.5
  Constant3 : Constant  Value=51544.5
  Sum : Sum  Inputs=+--
  MJD2000 : Outport
  wires:
  Constant3/1 -> Sum/3
  Constant1/1 -> Sum/2
  JD/1 -> Sum/1
  Sum/1 -> MJD2000/1

== system assignment_R2018A/On-Board Computer/Attitude Determination/Kinematics/LVLH/Full Orbital Dynamics ==
  mu : Inport
  Initial Condition (kep) : Inport  Port=2
  Compute R and V of reference orbit : Subsystem
  MATLAB Function : MATLAB Function  TreatAsAtomicUnit=on
  A_LN : Outport
  wires:
  mu/1 -> Compute R and V of reference orbit/1(mu)
  Initial Condition (kep)/1 -> Compute R and V of reference orbit/2(Initial Conditions)
  Compute R and V of reference orbit/1(r) -> MATLAB Function/1(r)
  MATLAB Function/1(A_LN) -> A_LN/1
  Compute R and V of reference orbit/2(r_dot) -> MATLAB Function/2(r_dot)

== system assignment_R2018A/On-Board Computer/Attitude Determination/Kinematics/Quaternions/Quaternions ==
  "q_0 " : Inport
  ω_bn : Inport  Port=2
  Integrator2 : Integrator  InitialConditionSource=external  InitialCondition=q_0
  Quaternion Kinematics : MATLAB Function  TreatAsAtomicUnit=on
  quaternions : Outport
  wires:
  Integrator2/1 -> Quaternion Kinematics/1(q), quaternions/1  "q"
  Quaternion Kinematics/1(q_dot) -> Integrator2/1  "dq"
  ω_bn/1 -> Quaternion Kinematics/2(omega)  "ω_b"
  "q_0 "/1 -> Integrator2/2

== system assignment_R2018A/True Error/Body\LVLH Difference/LVLH/Full Orbital Dynamics/Compute R and V of reference orbit ==
  mu : Inport
  Initial Conditions : Inport  Port=2
  Initial Position : Subsystem
  Initial Velocity : Subsystem
  Integrator : Integrator  InitialConditionSource=external  InitialCondition=[r,v]=kep2car(kep,mu);  ContinuousStateAttributes='velocity'
  Integrator2 : Integrator  InitialConditionSource=external  InitialCondition=[r,v]=kep2car(kep,mu);  ContinuousStateAttributes='position'
  Orbital Dynamics : MATLAB Function  TreatAsAtomicUnit=on
  r : Outport
  r_dot : Outport  Port=2
  wires:
  Initial Conditions/1 -> Initial Position/2(Initial Conditions), Initial Velocity/2(Initial Conditions)
  Initial Position/1(r_0) -> Integrator2/2
  Initial Velocity/1(r_dot_0) -> Integrator/2
  Orbital Dynamics/1(r_dot_dot) -> Integrator/1
  Integrator/1 -> r_dot/1, Integrator2/1
  mu/1 -> Initial Position/1(mu), Initial Velocity/1(mu), Orbital Dynamics/2(mu)
  Integrator2/1 -> Orbital Dynamics/1(r), r/1

== system assignment_R2018A/On-Board Computer/Attitude Determination/Kinematics/LVLH/Full Orbital Dynamics/Compute R and V of reference orbit ==
  mu : Inport
  Initial Conditions : Inport  Port=2
  Discrete-Time Integrator : DiscreteIntegrator  IntegratorMethod=Integration: Trapezoidal  InitialConditionSource=external  SampleTime=-1  ICPrevOutput=DiscIntNeverNeededParam  ICPrevScaledInput=DiscIntNeverNeededParam
  Discrete-Time Integrator1 : DiscreteIntegrator  IntegratorMethod=Integration: Trapezoidal  InitialConditionSource=external  SampleTime=-1  ICPrevOutput=DiscIntNeverNeededParam  ICPrevScaledInput=DiscIntNeverNeededParam
  Initial Position : Subsystem
  Initial Velocity : Subsystem
  Orbital Dynamics : MATLAB Function  TreatAsAtomicUnit=on
  r : Outport
  r_dot : Outport  Port=2
  wires:
  Initial Conditions/1 -> Initial Position/2(Initial Conditions), Initial Velocity/2(Initial Conditions)
  Initial Position/1(r_0) -> Discrete-Time Integrator1/2
  Initial Velocity/1(r_dot_0) -> Discrete-Time Integrator/2
  Orbital Dynamics/1(r_dot_dot) -> Discrete-Time Integrator/1
  Discrete-Time Integrator/1 -> Discrete-Time Integrator1/1, r_dot/1
  mu/1 -> Initial Position/1(mu), Initial Velocity/1(mu), Orbital Dynamics/2(mu)
  Discrete-Time Integrator1/1 -> Orbital Dynamics/1(r), r/1

== system assignment_R2018A/True Error/Body\LVLH Difference/LVLH/Full Orbital Dynamics/Compute R and V of reference orbit/Initial Position ==
  mu : Inport
  Initial Conditions : Inport  Port=2
  MATLAB Function2 : MATLAB Function  TreatAsAtomicUnit=on
  r_0 : Outport
  wires:
  MATLAB Function2/1(r_0) -> r_0/1
  mu/1 -> MATLAB Function2/2(mu)
  Initial Conditions/1 -> MATLAB Function2/1(kep)

== system assignment_R2018A/True Error/Body\LVLH Difference/LVLH/Full Orbital Dynamics/Compute R and V of reference orbit/Initial Velocity ==
  mu : Inport
  Initial Conditions : Inport  Port=2
  MATLAB Function1 : MATLAB Function  TreatAsAtomicUnit=on
  r_dot_0 : Outport
  wires:
  MATLAB Function1/1(r_dot_0) -> r_dot_0/1
  mu/1 -> MATLAB Function1/2(mu)
  Initial Conditions/1 -> MATLAB Function1/1(kep)

== system assignment_R2018A/On-Board Computer/Attitude Determination/Kinematics/LVLH/Full Orbital Dynamics/Compute R and V of reference orbit/Initial Position ==
  mu : Inport
  Initial Conditions : Inport  Port=2
  MATLAB Function2 : MATLAB Function  TreatAsAtomicUnit=on
  r_0 : Outport
  wires:
  MATLAB Function2/1(r_0) -> r_0/1
  mu/1 -> MATLAB Function2/2(mu)
  Initial Conditions/1 -> MATLAB Function2/1(kep)

== system assignment_R2018A/On-Board Computer/Attitude Determination/Kinematics/LVLH/Full Orbital Dynamics/Compute R and V of reference orbit/Initial Velocity ==
  mu : Inport
  Initial Conditions : Inport  Port=2
  MATLAB Function1 : MATLAB Function  TreatAsAtomicUnit=on
  r_dot_0 : Outport
  wires:
  MATLAB Function1/1(r_dot_0) -> r_dot_0/1
  mu/1 -> MATLAB Function1/2(mu)
  Initial Conditions/1 -> MATLAB Function1/1(kep)

== matlab function assignment_R2018A/Attitude Matrix/Kinematics: Euler Angles/MATLAB Function ==
  data: phi_dot output; tetha_dot output; psi_dot output; w input; tetha input; psi input
function [phi_dot,tetha_dot, psi_dot] = euler_eqtns(w, tetha, psi)

% Euler rotations (sequence 321)
phi_dot = 1/cos(tetha)*(w(2)*sin(psi) + w(3)*cos(psi));
tetha_dot = (w(2)*cos(psi)-w(3)*sin(psi));
psi_dot = w(1) + 1/cos(tetha)*(w(2)*sin(tetha)*sin(psi) + w(3)*sin(tetha)*cos(psi)); 

end

== matlab function assignment_R2018A/Attitude Matrix/MATLAB Function ==
  data: w input; w_cross output
function w_cross  = assembly_w_cross(w)

w_cross = [0, -w(3), w(2);
           w(3), 0, -w(1);
          -w(2), w(1), 0];

== matlab function assignment_R2018A/Attitude Matrix/MATLAB Function1 ==
  data: u input; y output
function y = ortonormalize(u)
%#codegen
% Ortonormalize a matrix.
% Reference : Lecture 7, Slide 5 SADC Polimi

y = u.*3/2 - u*u'*(u./2);

y = u;

end

== matlab function assignment_R2018A/Attitude Matrix/Quaternions/Quaternion Kinematics ==
  data: q input size=4; q_dot output size=4; omega input size=3
function q_dot = quat_kin(q, omega)

qnorm = sqrt(q(1)^2 + q(2)^2 + q(3)^2 + q(4)^2);
q = q./qnorm;

W = [ q(4) -q(3)  q(2) ;
      q(3)  q(4) -q(1) ;
     -q(2)  q(1)  q(4) ; 
     -q(1) -q(2) -q(3)];

q_dot = 0.5 * W * omega;

== matlab function assignment_R2018A/Disturbance Torques/Areodynamic Drag Torque Calculator /MATLAB Function ==
  data: vw_rel_body input; vw_rel input; drag_torque output; A_i input; dim input; rho input; C_d input
function drag_torque   = aerodrag(vw_rel_body,vw_rel,A_i,dim,rho, C_d)

% Velocity is in km/s, we need it in m/s
vw_rel_body = vw_rel_body .* 1e3;
vw_rel = vw_rel .* 1e3;

% Define normal vectors
n_1 = [1 0 0];
n_2 = [0 1 0];
n_3 = [0 0 1];
n_4 = [-1 0 0];
n_5 = [0 -1 0];
n_6 = [0 0 -1];

% Dimensions
w = dim(1);
l = dim(2);
h = dim(3);

% Sections
A_i_1 = A_i(1);
A_i_2 = A_i(2);
A_i_3 = A_i(3);
A_i_4 = A_i(1);
A_i_5 = A_i(2);
A_i_6 = A_i(3);

% Distance between the center of pressure and the center of mass 0.1*rcg
r_1 = [h/2 0.1 0.1];
r_2 = [0.2 l/2 0.2];
r_3 = [0.4 0.4 w/2];
r_4 = [-h/2 0.1 0.1];
r_5 = [0.2 -l/2 0.2];
r_6 = [0.4 0.4 -w/2];

% Compute Aerodynamic Torque : reference Fundamentals of Spacecraft
% Dynamics and Control pag. 108
% Compute the dynamic pressure
dynamic_pressure = -0.5*rho*norm(vw_rel)*vw_rel_body;

% Compute torque due to the aerodynamic force only on face wetted by air
% If dot(n_1,vw_rel_body/norm(vw_rel_body)) >=0 then the face is wetted
% othewise no.
if dot(n_1,vw_rel_body/norm(vw_rel)) >= 0
    F_aero_1 = dynamic_pressure * C_d * A_i_1 * dot(n_1,vw_rel_body)/norm(vw_rel);
    T_aero_1 = cross(r_1,F_aero_1);
else
    T_aero_1 = [0 0 0];
end

if dot(n_2,vw_rel_body/norm(vw_rel)) >= 0
    F_aero_2 = dynamic_pressure * C_d * A_i_2 * dot(n_2,vw_rel_body)/norm(vw_rel);
    T_aero_2 = cross(r_2,F_aero_2);
else
    T_aero_2 = [0 0 0];
end

if dot(n_3,vw_rel_body/norm(vw_rel)) >= 0
    F_aero_3 = dynamic_pressure * C_d * A_i_3 * dot(n_3,vw_rel_body)/norm(vw_rel);
    T_aero_3 = cross(r_3,F_aero_3);
else
    T_aero_3 = [0 0 0];
end

if dot(n_4,vw_rel_body/norm(vw_rel)) >= 0
    F_aero_4 = dynamic_pressure * C_d * A_i_4 * dot(n_4,vw_rel_body)/norm(vw_rel);
    T_aero_4 = cross(r_4,F_aero_4);
else
    T_aero_4 = [0 0 0];
end

if dot(n_5,vw_rel_body/norm(vw_rel)) >= 0
    F_aero_5 = dynamic_pressure * C_d * A_i_5 * dot(n_5,vw_rel_body)/norm(vw_rel);
    T_aero_5 = cross(r_5,F_aero_5);
else
    T_aero_5 = [0 0 0];
end

if dot(n_6,vw_rel_body/norm(vw_rel)) >= 0
    F_aero_6 = dynamic_pressure * C_d * A_i_6 * dot(n_6,vw_rel_body)/norm(vw_rel);
    T_aero_6 = cross(r_6,F_aero_6);
else
    T_aero_6 = [0 0 0];
end

% Sum drag on all the surface
drag_torque = [T_aero_1 + T_aero_2 + T_aero_3 + T_aero_4 + T_aero_5 + T_aero_5 + T_aero_6]';

end

== matlab function assignment_R2018A/On-Board Computer/Pointing Control/Quaternion Feedback Control/Command Quaternion/MATLAB Function ==
  data: A input; quat output
function quat = attToQuat( A )
%   Converts the attitude matrix A to a quaternion vector using a modification 
%   of the "Shepperd's Algorithm"
%
%   quat = attToQuat( A )
%
%   The attitude matrix A represents the rotational matrix from the inertial
%   reference frame to the body frame of the vehicle.
%   The quaternion (quat) will be returned as a 4-by-1 vector with the scalar
%   element as the fourth component.
%
%   References:
%	[1] Markley, F. Landis. "Unit quaternion from rotation matrix." 
%       Journal of guidance, control, and dynamics 31.2 (2008): 440.

vector = [A(1,1), A(2,2), A(3,3), trace(A)];
[M, i] = max(vector);

switch i
    case 1
        q = [ 1 + A(1,1) - A(2,2) - A(3,3);
            A(1,2) + A(2,1);
            A(1,3) + A(3,1);
            A(2,3) - A(3,2)];
        
    case 2
        q = [A(2,1) + A(1,2);
            1 + A(2,2) - A(3,3) - A(1,1);
            A(2,3) + A(3,2);
            A(3,1) - A(1,3)];
        
    case 3
        q = [A(3,1) + A(1,3);
            A(3,2) + A(2,3);
            1 + A(3,3) - A(1,1) - A(2,2);
            A(1,2) - A(2,1)];
        
    case 4
        q = [A(2,3) - A(3,2);
            A(3,1) - A(1,3);
            A(1,2) - A(2,1);
            1 + A(1,1) + A(2,2) + A(3,3);];
        
    otherwise
        error('Check the Attitude matrix');
end

quat = q / norm(q);

== matlab function assignment_R2018A/Disturbance Torques/Areodynamic Drag Torque Calculator /MATLAB Function1 ==
  data: r_LVLH input; rho output; R_e input
function rho = density_calculator(r_LVLH,R_e)
%#codegen
% Exponential model for computing density

h = norm(r_LVLH') - R_e;


H = 0;
h0 = 0;
rho_0 = 0; 
rho = 0;

if h > 200 && h <= 250
    H = 38.5;
    h0 = 200;
    rho_0 = 2.780e-10;
elseif h > 250 && h <= 300
    H = 46.9;
    h0 = 250;
    rho_0 = 7.248e-11;
elseif h > 300 && h <= 350
    H = 52.5;
    h0 = 300;
    rho_0 = 2.418e-11;
elseif h > 350 && h <= 400
    H = 56.4;
    h0 = 350;
    rho_0 = 9.158e-12;
elseif h > 400 && h <= 450
    H = 59.4;
    h0 = 400;
    rho_0 = 3.725e-12;
elseif h > 450 && h <= 500
    H = 62.2;
    h0 = 450;
    rho_0 = 1.585e-12;
elseif h > 500 && h <= 600
    H = 65.8;
    h0 = 500;
    rho_0 = 6.967e-13;
elseif h > 600 && h <= 700
    H = 79.0;
    h0 = 600;
    rho_0 = 1.454e-13;
elseif h > 700 && h <= 800
    H = 109.0;
    h0 = 700;
    rho_0 = 3.614e-14;
elseif h > 800 && h <= 900
    H = 164.0;
    h0 = 800;
    rho_0 = 1.170e-14;
elseif h > 900 && h < 1000
    H = 225.0;
    h0 = 900;
    rho_0 = 5.245e-15;
elseif h > 1000 
    H = 260.0;
    h0 = 1000;
    rho_0 = 3.019e-15;
end

rho = rho_0*exp(-(h-h0)/H);

== matlab function assignment_R2018A/True Error/Angular velocity of the orbital pointing frame/MATLAB Function ==
  data: w_ln_cross input; w_ln output
function w_ln = w_component_extractor(w_ln_cross)

w_1 = w_ln_cross(3,2);
w_2 = w_ln_cross(1,3);
w_3 = w_ln_cross(2,1);

w_ln = [w_1, w_2, w_3]';
end

== matlab function assignment_R2018A/True Error/Body\LVLH Difference/LVLH/Full Orbital Dynamics/Compute R and V of reference orbit/Initial Position/MATLAB Function2 ==
  data: r_0 output; kep input; mu input
function r_0  = kep2car(kep,mu)

% Using kep2car function to find position and velocity at initial condition
[r_0,~]=kep2car(kep,mu);

end

== matlab function assignment_R2018A/True Error/Body\LVLH Difference/LVLH/Full Orbital Dynamics/Compute R and V of reference orbit/Initial Velocity/MATLAB Function1 ==
  data: r_dot_0 output; kep input; mu input
function r_dot_0  = kep2car(kep,mu)

% Using kep2car function to find velocity at initial condition
[~,r_dot_0]=kep2car(kep,mu);

end

== matlab function assignment_R2018A/True Error/Body\LVLH Difference/LVLH/Full Orbital Dynamics/Compute R and V of reference orbit/Orbital Dynamics ==
  data: r input; r_dot_dot output; mu input
function r_dot_dot  = orbit_equation(r,mu)

r_dot_dot = -(mu/norm(r)^3)*r;

end

== matlab function assignment_R2018A/True Error/Body\LVLH Difference/LVLH/Full Orbital Dynamics/MATLAB Function ==
  data: r input; A_LN output; r_dot input
function A_LN = assembly_A_LN(r,r_dot)
% This M-Function builds an LVLH frame from a position vector and a 
% velocity vector

r = r';
r_dot = r_dot';

o_1 = - r/norm(r);                                      % Points toward the Earth, aligned with S/C - Earth direction (x)
o_3 = - (cross(r,r_dot))/(norm(cross(r,r_dot)));         % Points in the direction of angular momentum vector (z)
o_2 = cross(o_3,o_1);                                   % Points into the direction of the motion (y)

A_LN = [o_1; o_2; o_3];

end
